simulink model "task_1_sim"  (R2023a)
settings: Solver=VariableStepAuto  StartTime=0.0  StopTime=10  MaxStep=0.0001  RelTol=1e-5
undefined symbols (not defined in the file): A, B, K, K1, x0
settings Model: Creator=user  LastModifiedBy=user

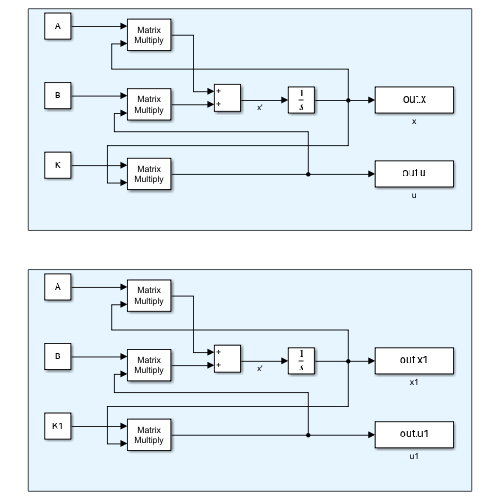
[thumbnail: Simulink's stored preview of the top-level diagram]
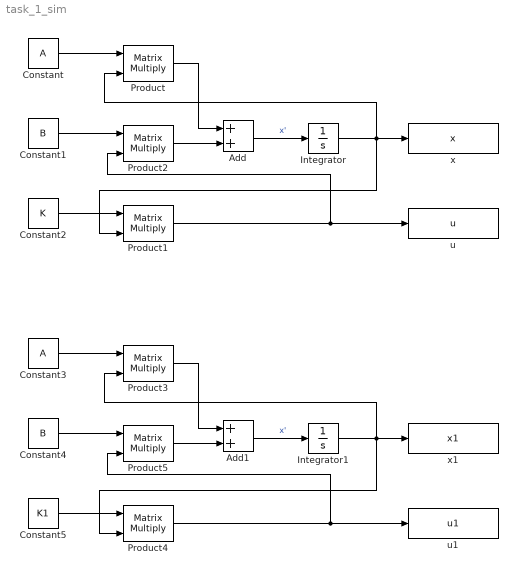
== system task_1_sim ==
  Add : Sum
  Add1 : Sum
  Constant : Constant  Value=A
  Constant1 : Constant  Value=B  VectorParams1D=off
  Constant2 : Constant  Value=K  VectorParams1D=off
  Constant3 : Constant  Value=A
  Constant4 : Constant  Value=B  VectorParams1D=off
  Constant5 : Constant  Value=K1  VectorParams1D=off
  Integrator : Integrator  InitialCondition=x0
  Integrator1 : Integrator  InitialCondition=x0
  Product{,1..5} (6 alike) : Product  Multiplication=Matrix(*)
  u : ToWorkspace  VariableName=u  SaveFormat=Timeseries  SampleTime=-1
  u1 : ToWorkspace  VariableName=u1  SaveFormat=Timeseries  SampleTime=-1
  x : ToWorkspace  VariableName=x  SaveFormat=Timeseries  SampleTime=-1
  x1 : ToWorkspace  VariableName=x1  SaveFormat=Timeseries  SampleTime=-1
  wires:
  Constant2/1 -> Product1/1
  Integrator/1 -> Product/2, x/1, Product1/2
  Constant/1 -> Product/1
  Product1/1 -> u/1, Product2/2
  Constant1/1 -> Product2/1
  Product2/1 -> Add/2
  Product/1 -> Add/1
  Add/1 -> Integrator/1  "x'"
  Product3/1 -> Add1/1
  Add1/1 -> Integrator1/1  "x'"
  Product5/1 -> Add1/2
  Constant5/1 -> Product4/1
  Constant3/1 -> Product3/1
  Product4/1 -> u1/1, Product5/2
  Constant4/1 -> Product5/1
  Integrator1/1 -> Product3/2, x1/1, Product4/2
